simulink model "vd_controller_E9"  (R2017b)
settings: configuration reference "E9_ECU_Configuration" (kept outside this file)
undefined symbols (not defined in the file or in its folder): activate_TC_forMinimal_pTC, ConstantSlipPercent_XCP_pTC, DifferentTorqueFrontAxis_tc, disable_9D_front, disable_9D_rear, disable_slipanglesensor, DiscIntNeverNeededParam, Fz0, lambda_mux_switch_over_XCP_pTC, lambda_mux_XCP_pTC, Lyap_kp_switch_over_XCP_pTC, Lyap_kp_XCP_pTC, Lyap_p, Lyap_TCint, LyapDiscFilter, lyapFilterCoeff_switch_over_XCP_pTC, lyapFilterCoeff_XCP_pTC, mask_SelectInput_pGL, p_Dx1, p_Dx2, Slip_switch_over_XCP_pTC, Sq_PosBadGradient, Sq_PosIsFrozen, Sq_PosOutOfBounds, tire_r_dyn, velLimitInput_switch_over_XCP_pTC, velLimitInput_XCP_pTC, WheelInertia
libraries: SignalProcessingLib x37, simulink x30, hdlsllib x3
(part 1 of 2)
settings Model: DataDictionary=dd_MainControl_E9.sldd  ExplicitPartitioning=on  Creator=chwit  LastModifiedBy=gt-testing
settings Model: ModifiedComment=|
  | schwa -- Fri Mar 02 10:09:33 2018 -- Version 1.53
  | Switched names of ControlAllocation, minimal Version active
settings Model: ModifiedHistory=|
  | schwa -- Fri Mar 02 10:09:33 2018 -- Version 1.53
  | Switched names of ControlAllocation, minimal Version active
  | 
  | schwa -- Fri Mar 02 10:09:33 2018 -- Version 1.53
  | Switched names of ControlAllocation, minimal Version active
  | 
  | schwa -- Fri Mar 02 01:32:20 2018 -- Version 1.52
  | cosmetic changes, adjusted ports
  | 
  | schwa -- Fri Mar 02 01:28:29 2018 -- Version 1.51
  | 
  | schwa -- Fri Mar 02 01:26:02 2018 -- Version 1.50
  | integrated new FF
  | 
  | 
  | chwit -- Fri Feb 23 19:55:57 2018 -- Version 1.49
  | 
  | chwit -- Fri Feb 23 07:06:27 2018 -- Version 1.48
  | Buildable but yet not flashable version of initial version of ControlSystem for E9 after function freeze v1
  | 
  | 
  | 
  | chwit -- Sun Feb 18 18:12:23 2018 -- Version 1.20
  | 
  | chwit -- Sun Feb 18 18:12:23 2018 -- Version 1.20
  | 
  | chwit -- Sun Feb 18 18:02:59 2018 -- Version 1.19
  | 
  | chwit -- Sun Feb 18 17:57:29 2018 -- Version 1.18
  | Saving
  | 
  | 
  | chwit -- Sun Feb 18 17:09:51 2018 -- Version 1.17
  | Saving
  | 
  | chwit -- Sun Feb 18 17:09:04 2018 -- Version 1.16
  | Just for saving purposes
  | 
  | chwit -- Sun Feb 18 14:38:44 2018 -- Version 1.15
  | YawMoment -> YawAcc corrected
  | 
  | 
  | chwit -- Sun Feb 18 12:57:57 2018 -- Version 1.14
  | Function freeze and new structure
  | 
  | 
  | chwit -- Sun Feb 18 12:51:11 2018 -- Version 1.13
  | Changes made due to function freeze and new structure
  | 
  | 
  | chwit -- Sun Feb 18 11:51:16 2018 -- Version 1.11
  | Implemented Manual Mode
  | 
  | chwit -- Sun Feb 18 11:51:16 2018 -- Version 1.11
  | Implemented Manual Mode
  | 
  | Marko -- Sat Feb 17 23:21:38 2018 -- Version 1.10
  | Changed Subsystem ConvertToInverterSingals: Deleted Everything except kt-Kennlinie, added limit on TorqueRequest
  | 
  | added OverUndersteerCorrection between FF and CA, connected CA with temporary (dummy) signals until right signals are provided
  | schwa -- Wed Feb 14 10:07:50 2018 -- Version 1.9
  | 
  | rearranged signals
  | schwa -- Wed Feb 14 09:51:50 2018 -- Version 1.8
  | 
  | chwit -- Sat Jan 20 18:54:27 2018 -- Version 1.7
  | 
  | chwit -- Sat Jan 20 17:46:44 2018 -- Version 1.6
  | 
  | chwit -- Sat Jan 20 17:42:35 2018 -- Version 1.5
  | Initial version
settings ConfigSetRef: DDName=dd_MainControl_E9.sldd

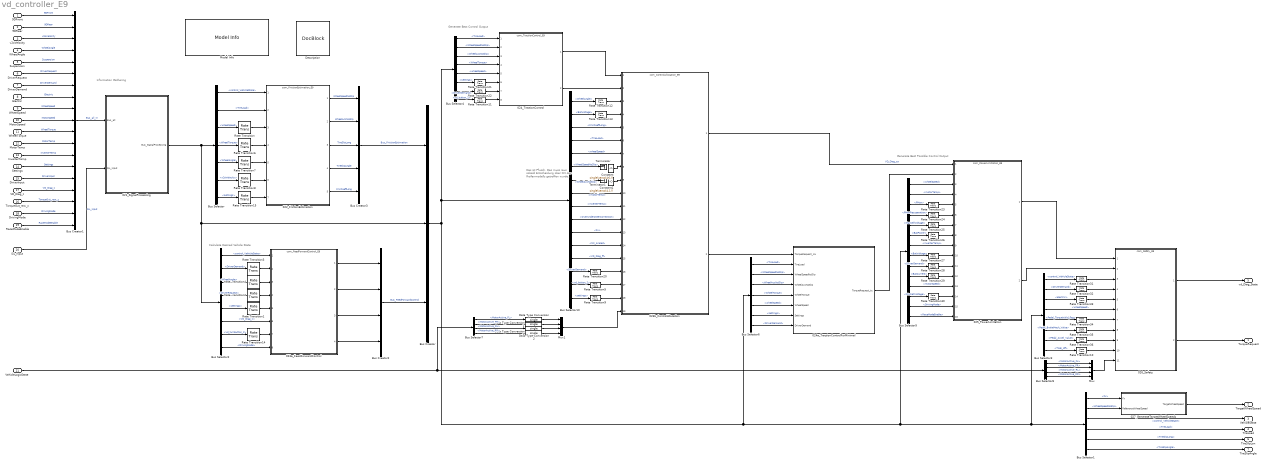
== system vd_controller_E9 ==
  note: Das ist Pfusch.
      | Das muss raus sobald
      | Entscheidung über Ort des
      |  Reifenmodells getroffen wurde.
  note: Information Gathering
  note: Calculate Desired Vehicle State
  note: Generate Best Control Output
  note: Generate Best Possible Control Output
  9DFront : Inport  OutDataTypeStr=Bus: control_9D
  9DRear : Inport  Port=2  OutDataTypeStr=Bus: control_9D
  v2oVelocity : Inport  Port=3  OutDataTypeStr=Bus: control_Velocity  SampleTime=0.004
  WheelAngle : Inport  Port=4  OutDataTypeStr=Bus: control_WheelAngle  SampleTime=0.01
  Suspension : Inport  Port=5  OutDataTypeStr=Bus: control_Suspension  SampleTime=0.01
  DriverRequest : Inport  Port=6  OutDataTypeStr=Bus: control_DriverRequest  SampleTime=0.01
  DriverDemand : Inport  Port=7  OutDataTypeStr=single  PortDimensions=1  SampleTime=0.01
  Electric : Inport  Port=8  OutDataTypeStr=Bus: control_Electric  SampleTime=0.002
  WheelSpeed : Inport  Port=9  OutDataTypeStr=single  PortDimensions=4  SampleTime=0.001
  MotorSpeed : Inport  Port=10  OutDataTypeStr=single  PortDimensions=[4 1]
  WheelTorque : Inport  Port=11  OutDataTypeStr=single  PortDimensions=4  SampleTime=0.001
  MotorTemp : Inport  Port=12  OutDataTypeStr=single  PortDimensions=[4 1]
  InverterTemp : Inport  Port=13  PortDimensions=[4 1]
  Settings : Inport  Port=14  OutDataTypeStr=Bus: control_Settings  SampleTime=0.1
  DriverInput : Inport  Port=15  OutDataTypeStr=Bus: control_DriverInput  SampleTime=0.1
  TorqueOut_raw_z : Inport  Port=16  OutDataTypeStr=single  PortDimensions=4
  VD_Diag_z : Inport  Port=17  OutDataTypeStr=uint16
  DrivingMode : Inport  Port=18  OutDataTypeStr=single  PortDimensions=1
  RaceModeEnable : Inport  Port=19  OutDataTypeStr=boolean
  SiL_Input : Inport  Port=20  OutDataTypeStr=Bus: control_SiL_Input
  VehicleLogicState : Inport  Port=21  OutDataTypeStr=Bus: control_VehicleLogicState
  021_SignalProcessing : Subsystem
  022_FrictionEstimation : ModelReference  ModelNameDialog=com_FrictionEstimation_E9.slx  SimulationMode=Normal  ModelReferenceVersion=1.57
  023a_FeedForwardControl : ModelReference  ModelNameDialog=com_FeedForwardControl_E9.slx  SimulationMode=Normal  ModelReferenceVersion=1.225
  023b_ControlAllocation : ModelReference  ModelNameDialog=com_ControlAllocation_E9.slx  SimulationMode=Normal  ModelReferenceVersion=1.346
  024_TractionControl : ModelReference  ModelNameDialog=com_TractionControl_E9.slx  SimulationMode=Normal  ModelReferenceVersion=1.68
  024a_TractionControlForMinimal : Subsystem
  025_PowerLimitation : ModelReference  ModelNameDialog=com_PowerLimitation_E9.slx  SimulationMode=Normal  ModelReferenceVersion=1.208
  026_Safety : ModelReference  ModelNameDialog=com_Safety_E9.slx  SimulationMode=Normal  ModelReferenceVersion=1.81
  027_GenerateTargetWheelSpeeds : Subsystem
  Bus Creator : BusCreator  Inputs=3
  Bus Creator1 : BusCreator  Inputs=19
  Bus Creator2 : BusCreator  Inputs=4
  Bus Creator3 : BusCreator  Inputs=5
  Bus Selector : BusSelector  OutputSignals=control_VehicleState,TireLoad,wheelSpeed,WheelTorque,WheelAngle,v2oVelocity,settings
  Bus Selector1 : BusSelector  OutputSignals=Bus_FeedForwardControl.Fx,Bus_FrictionEstimation.WheelSpeedNoSlip,Bus_SignalProcessing.control_VehicleState,Bus_SignalProcessing.TireLoad,Bus_FrictionEstimation.TireSlipLong,Bus_FrictionEstimation.TireSlipAngle
  Bus Selector10 : BusSelector  OutputSignals=Bus_SignalProcessing.WheelAngle,Bus_SignalProcessing.electric.BatVoltage,Bus_FrictionEstimation.FricCoeffLong,Bus_SignalProcessing.TireLoad,Bus_SignalProcessing.wheelSpeed,Bus_FrictionEstimation.WheelSpeedNoSlip,Bus_FrictionEstimation.WheelAccNoSlip,Bus_SignalProcessing.motorTemp,Bus_SignalProcessing.inverterTemp,Bus_FeedForwardControl.OverUndersteerCorrection,Bus_FeedForwardControl.Fx,Bus_FeedForwardControl.Mz_scaled,Bus_FeedForwardControl.VD_Diag_ff,Bus_SignalProcessing.DriverDemand,Bus_SignalProcessing.HMI_DriverNotice.vd_button_2,Bus_SignalProcessing.settings
  Bus Selector2 : BusSelector  OutputSignals=control_VehicleState,DriverDemand,WheelAngle,DriverRequest,settings,VD_Diag_z,HMI_DriverNotice.vd_turnbutton_2,HMI_DriverNotice.DrivingMode
  Bus Selector3 : BusSelector  OutputSignals=Bus_SignalProcessing.control_VehicleState,Bus_SignalProcessing.DriverDemand,Bus_SignalProcessing.electric,Bus_SignalProcessing.wheelSpeed,Bus_SignalProcessing.DriverRequest.Pedal_TorqueValid_flag,Bus_SignalProcessing.DriverRequest.Pedal_BrakeMech_Value,Bus_SignalProcessing.DriverRequest.Pedal_Accel_Value,Bus_SignalProcessing.settings.TWB_off
  Bus Selector4 : BusSelector  OutputSignals=Bus_SignalProcessing.TireLoad,Bus_FrictionEstimation.WheelSpeedNoSlip,Bus_FrictionEstimation.WheelAccNoSlip,Bus_SignalProcessing.WheelTorque,Bus_SignalProcessing.wheelSpeed,Bus_SignalProcessing.settings,Bus_SignalProcessing.DriverDemand,Bus_SignalProcessing.HMI_DriverNotice.vd_button_2
  Bus Selector5 : BusSelector  OutputSignals=Bus_SignalProcessing.wheelSpeed,Bus_SignalProcessing.motorTemp,Bus_SignalProcessing.settings.PMax,Bus_SignalProcessing.settings.PMaxRecuperation,Bus_SignalProcessing.electric.MaxCellVoltage,Bus_SignalProcessing.electric.BatPower,Bus_SignalProcessing.inverterTemp,Bus_SignalProcessing.electric.BatVoltage,Bus_SignalProcessing.DriverDemand,Bus_SignalProcessing.electric.BatCurrent,Bus_SignalProcessing.motorSpeed,Bus_SignalProcessing.electric.MinCellVoltage,Bus_SignalProcessing.HMI_DriverNotice.DrivingMode,Bus_SignalProcessing.RaceModeEnable
  Bus Selector6 : BusSelector  OutputSignals=Bus_SignalProcessing.TireLoad,Bus_FrictionEstimation.WheelSpeedNoSlip,Bus_FrictionEstimation.WheelAccNoSlip,Bus_SignalProcessing.WheelTorque,Bus_SignalProcessing.wheelSpeed,Bus_SignalProcessing.settings,Bus_SignalProcessing.DriverDemand
  Bus Selector7 : BusSelector  OutputSignals=MotorActive_FL,MotorActive_FR,MotorActive_RL,MotorActive_RR
  Bus Selector8 : BusSelector  OutputSignals=MotorActive_FL,MotorActive_FR,MotorActive_RL,MotorActive_RR
  Constant : Constant  Value=single(zeros(4,1))
  Constant1 : Constant  Value=single(zeros(4,1))
  Data Type Conversion{,1..3} (4 alike) : DataTypeConversion  OutDataTypeStr=single
  Description : simulink/Model-Wide Utilities/DocBlock  DocumentType=Text
      content=|
      | Beschreibung:
      |
      | Schlupfsollwert wird über Settings-Protokoll vorgegeben. Wird entsprechend mit Vorzeichen Torque-Request verrechnet.
      | Desgin-Parameter sind Lyap_kp (nützlich, linearer Faktor) und Lyap_p (nicht so nützlich, Potenz -> sollte ungerade sein (nicht ganz sicher)).
      |
      | I-Anteil mit Anti-WindUp zur Verbesserung Regler und Stellgrößenbeschränkung vorzubeugen.
      |
      | Tiefpassfilter (PT1) zur Verminderung von Schwingungen.
      |
      | Lambda_mux ist der Einstellparameter für den Reibwert, mit dem das SetUp stark verändert werden kann.
      |
      | Multiport-Switches zur Auswahl diverser Ansätze für die Traktionskontrolle bzw. zur Abschaltung.
      |
      | Adaptive_RG Schlupfgeschw.: adaptiver Regler mit Reibwerschätzer, schätzt Reibwert und regelt entsprechend Schlupf
      |     -> hat nicht wirklich funktioniert, Schätzen war wohl schon scheiße, Konzept fragwürdig
      |
      | LQRI: Linearisierter Lyap. Regler mit diversen Betriebspunkten (Gain-Scheduling), ähnliche Gleichungen wie Lyap
      |     -> durch Linearisierung etwas schlechter als Lyap
  Model Info : simulink/Model-Wide Utilities/Model Info  Frame=on  DisplayStringWithTags=|  HorizontalTextAlignment=Center  LeftAlignmentValue=0.5
      | Model Name: %<ModelName>
      | Responsible: Christian Witte
      | 
      | Last modified by: %<LastModifiedBy>
      | Last modified: %<LastModificationDate>
      | Current Version: %<ModelVersion>
  Mux : Mux
  Mux1 : Mux
  Rate Transition{,1..4,6..8,14..15} (10 alike) : RateTransition  Deterministic=off  OutPortSampleTime=0.002
  Rate Transition{5,9..13,20..36} (23 alike) : RateTransition  Deterministic=off  OutPortSampleTime=0.001
  Terminator : Terminator
  Terminator1 : Terminator
  TorqueRequest : Outport  OutDataTypeStr=single  PortDimensions=4
  TargetWheelSpeed : Outport  Port=2  OutDataTypeStr=single  PortDimensions=4
  VehicleState : Outport  Port=3  OutDataTypeStr=Bus: control_VehicleState
  TireLoad : Outport  Port=4  SignalName=TireLoad  OutDataTypeStr=single  PortDimensions=4
  vd_Diag_State : Outport  Port=5  OutDataTypeStr=uint16
  TireSlipLon : Outport  Port=6  OutDataTypeStr=single  PortDimensions=4
  TireSlipAngle : Outport  Port=7  OutDataTypeStr=single  PortDimensions=4
  wires:
  022_FrictionEstimation/3 -> Bus Creator3/3  "TireSlipLong"
  Bus Selector/2 -> 022_FrictionEstimation/2  "<TireLoad>"
  022_FrictionEstimation/2 -> Bus Creator3/2  "WheelAccNoSlip"
  Bus Selector/3 -> Rate Transition/1  "<wheelSpeed>"
  Bus Selector/1 -> 022_FrictionEstimation/1  "<control_VehicleState>"
  022_FrictionEstimation/1 -> Bus Creator3/1  "WheelSpeedNoSlip"
  Bus Creator3/1 -> Bus Creator/1  "Bus_FrictionEstimation"
  022_FrictionEstimation/4 -> Bus Creator3/4  "TireSlipAngle"
  025_PowerLimitation/1 -> 026_Safety/1
  023a_FeedForwardControl/4 -> Bus Creator2/4
  023b_ControlAllocation/1 -> 025_PowerLimitation/1  "VD_Diag_ca"
  Bus Creator1/1 -> 021_SignalProcessing/1(Bus_all)  "Bus_all_in"
  Bus Creator2/1 -> Bus Creator/3  "Bus_FeedForwardControl"
  021_SignalProcessing/1(Bus_SignalProcessing) -> Bus Selector/1, Bus Creator/2, Bus Selector2/1
  023a_FeedForwardControl/1 -> Bus Creator2/1
  023a_FeedForwardControl/3 -> Bus Creator2/3
  022_FrictionEstimation/5 -> Bus Creator3/5  "FricCoeffLong"
  Bus Creator/1 -> Bus Selector10/1, Bus Selector4/1, Bus Selector6/1, Bus Selector5/1, Bus Selector3/1, Bus Selector1/1
  Bus Selector1/3 -> VehicleState/1  "<control_VehicleState>"
  Bus Selector1/4 -> TireLoad/1  "<TireLoad>"
  023a_FeedForwardControl/2 -> Bus Creator2/2
  023b_ControlAllocation/2 -> 024a_TractionControlForMinimal/1(TorqueRequest_ca)
  Bus Selector5/1 -> 025_PowerLimitation/3  "<wheelSpeed>"
  Bus Selector5/2 -> 025_PowerLimitation/4  "<motorTemp>"
  Bus Selector5/3 -> Rate Transition23/1  "<PMax>"
  Bus Selector5/4 -> Rate Transition24/1  "<PMaxRecuperation>"
  Bus Selector5/5 -> Rate Transition25/1  "<MaxCellVoltage>"
  Bus Selector5/6 -> Rate Transition26/1  "<BatPower>"
  Bus Selector5/7 -> 025_PowerLimitation/9  "<inverterTemp>"
  Bus Selector5/8 -> Rate Transition27/1  "<BatVoltage>"
  Bus Selector5/9 -> Rate Transition28/1  "<DriverDemand>"
  Bus Selector3/1 -> Rate Transition31/1  "<control_VehicleState>"
  Bus Selector3/2 -> Rate Transition32/1  "<DriverDemand>"
  Bus Selector3/3 -> Rate Transition33/1  "<electric>"
  Bus Selector3/4 -> 026_Safety/6  "<wheelSpeed>"
  Bus Selector3/5 -> Rate Transition34/1  "<Pedal_TorqueValid_flag>"
  025_PowerLimitation/2 -> 026_Safety/2
  Bus Selector10/1 -> Rate Transition12/1  "<WheelAngle>"
  Bus Selector10/2 -> Rate Transition13/1  "<BatVoltage>"
  Bus Selector10/3 -> 023b_ControlAllocation/5  "<FricCoeffLong>"
  Bus Selector10/4 -> 023b_ControlAllocation/6  "<TireLoad>"
  Bus Selector10/5 -> 023b_ControlAllocation/7  "<wheelSpeed>"
  Bus Selector10/8 -> 023b_ControlAllocation/10  "<motorTemp>"
  Bus Selector10/9 -> 023b_ControlAllocation/11  "<inverterTemp>"
  Bus Selector10/10 -> 023b_ControlAllocation/12  "<OverUndersteerCorrection>"
  Bus Selector10/11 -> 023b_ControlAllocation/13  "<Fx>"
  026_Safety/2 -> TorqueRequest/1
  026_Safety/1 -> vd_Diag_State/1
  Bus Selector4/7 -> Rate Transition22/1  "<DriverDemand>"
  Bus Selector4/6 -> Rate Transition21/1  "<settings>"
  Bus Selector4/5 -> 024_TractionControl/5  "<wheelSpeed>"
  Bus Selector4/4 -> 024_TractionControl/4  "<WheelTorque>"
  Bus Selector4/3 -> 024_TractionControl/3  "<WheelAccNoSlip>"
  Bus Selector4/2 -> 024_TractionControl/2  "<WheelSpeedNoSlip>"
  Bus Selector4/1 -> 024_TractionControl/1  "<TireLoad>"
  Bus Selector10/13 -> 023b_ControlAllocation/15  "<VD_Diag_ff>"
  024_TractionControl/2 -> 023b_ControlAllocation/2
  024_TractionControl/1 -> 023b_ControlAllocation/1
  Constant/1 -> 023b_ControlAllocation/8
  Constant1/1 -> 023b_ControlAllocation/9
  Bus Selector10/6 -> Terminator/1  "<WheelSpeedNoSlip>"
  Bus Selector10/7 -> Terminator1/1  "<WheelAccNoSlip>"
  Bus Selector/4 -> Rate Transition6/1  "<WheelTorque>"
  Bus Selector/5 -> Rate Transition7/1  "<WheelAngle>"
  Bus Selector/6 -> Rate Transition8/1  "<v2oVelocity>"
  9DFront/1 -> Bus Creator1/1  "9DFront"
  9DRear/1 -> Bus Creator1/2  "9DRear"
  v2oVelocity/1 -> Bus Creator1/3  "v2oVelocity"
  WheelAngle/1 -> Bus Creator1/4  "WheelAngle"
  Suspension/1 -> Bus Creator1/5  "Suspension"
  DriverRequest/1 -> Bus Creator1/6  "DriverRequest"
  DriverDemand/1 -> Bus Creator1/7  "DriverDemand"
  TorqueOut_raw_z/1 -> Bus Creator1/17  "TorqueOut_raw_z"
  Electric/1 -> Bus Creator1/8  "Electric"
  VD_Diag_z/1 -> Bus Creator1/16  "VD_Diag_z"
  WheelSpeed/1 -> Bus Creator1/9  "WheelSpeed"
  MotorSpeed/1 -> Bus Creator1/10  "MotorSpeed"
  WheelTorque/1 -> Bus Creator1/11  "WheelTorque"
  MotorTemp/1 -> Bus Creator1/12  "MotorTemp"
  InverterTemp/1 -> Bus Creator1/13  "InverterTemp"
  Settings/1 -> Bus Creator1/14  "Settings"
  DriverInput/1 -> Bus Creator1/15  "DriverInput"
  Bus Selector2/1 -> 023a_FeedForwardControl/1  "<control_VehicleState>"
  Bus Selector2/2 -> Rate Transition3/1  "<DriverDemand>"
  Bus Selector2/3 -> Rate Transition4/1  "<WheelAngle>"
  Bus Selector2/4 -> Rate Transition2/1  "<DriverRequest>"
  Bus Selector2/5 -> Rate Transition1/1  "<settings>"
  Bus Selector2/6 -> 023a_FeedForwardControl/6  "<VD_Diag_z>"
  Bus Selector5/10 -> Rate Transition29/1  "<BatCurrent>"
  Bus Selector3/6 -> Rate Transition35/1  "<Pedal_BrakeMech_Value>"
  Bus Selector3/7 -> Rate Transition36/1  "<Pedal_Accel_Value>"
  SiL_Input/1 -> 021_SignalProcessing/2(SiL_Input)  "SiL_Input"
  Bus Selector10/14 -> Rate Transition20/1  "<DriverDemand>"
  Bus Selector1/2 -> 027_GenerateTargetWheelSpeeds/2(ReferenceWheelSpeed)  "<WheelSpeedNoSlip>"
  027_GenerateTargetWheelSpeeds/1(TargetWheelSpeed) -> TargetWheelSpeed/1
  Bus Selector1/1 -> 027_GenerateTargetWheelSpeeds/1(Fx)  "<Fx>"
  024a_TractionControlForMinimal/1(TorqueRequest_tc) -> 025_PowerLimitation/2
  Bus Selector6/1 -> 024a_TractionControlForMinimal/2(TireLoad)  "<TireLoad>"
  Bus Selector6/2 -> 024a_TractionControlForMinimal/3(WheelSpeedNoSlip)  "<WheelSpeedNoSlip>"
  Bus Selector6/3 -> 024a_TractionControlForMinimal/4(WheelAccNoSlip)  "<WheelAccNoSlip>"
  Bus Selector6/4 -> 024a_TractionControlForMinimal/5(WheelTorque)  "<WheelTorque>"
  Bus Selector6/5 -> 024a_TractionControlForMinimal/6(WheelSpeed)  "<wheelSpeed>"
  Bus Selector6/6 -> 024a_TractionControlForMinimal/7(Settings)  "<settings>"
  Bus Selector6/7 -> 024a_TractionControlForMinimal/8(DriverDemand)  "<DriverDemand>"
  Bus Selector5/11 -> 025_PowerLimitation/13  "<motorSpeed>"
  VehicleLogicState/1 -> Bus Selector7/1, Bus Selector8/1
  Rate Transition4/1 -> 023a_FeedForwardControl/3
  Rate Transition1/1 -> 023a_FeedForwardControl/5
  Rate Transition2/1 -> 023a_FeedForwardControl/4
  Rate Transition3/1 -> 023a_FeedForwardControl/2
  Rate Transition/1 -> 022_FrictionEstimation/3
  Rate Transition6/1 -> 022_FrictionEstimation/4
  Rate Transition7/1 -> 022_FrictionEstimation/5
  Rate Transition8/1 -> 022_FrictionEstimation/6
  Rate Transition12/1 -> 023b_ControlAllocation/3
  Rate Transition13/1 -> 023b_ControlAllocation/4
  Rate Transition20/1 -> 023b_ControlAllocation/16
  Rate Transition21/1 -> 024_TractionControl/6
  Rate Transition22/1 -> 024_TractionControl/7
  Rate Transition23/1 -> 025_PowerLimitation/5
  Rate Transition24/1 -> 025_PowerLimitation/6
  Rate Transition26/1 -> 025_PowerLimitation/8
  Rate Transition25/1 -> 025_PowerLimitation/7
  Rate Transition27/1 -> 025_PowerLimitation/10
  Rate Transition28/1 -> 025_PowerLimitation/11
  Rate Transition29/1 -> 025_PowerLimitation/12
  Rate Transition30/1 -> 025_PowerLimitation/14
  Rate Transition31/1 -> 026_Safety/3
  Rate Transition32/1 -> 026_Safety/4
  Rate Transition33/1 -> 026_Safety/5
  Rate Transition34/1 -> 026_Safety/7
  Rate Transition35/1 -> 026_Safety/8
  Rate Transition36/1 -> 026_Safety/9
  Bus Selector8/1 -> Mux/1  "<MotorActive_FL>"
  Bus Selector8/2 -> Mux/2  "<MotorActive_FR>"
  Bus Selector8/3 -> Mux/3  "<MotorActive_RL>"
  Bus Selector8/4 -> Mux/4  "<MotorActive_RR>"
  Mux/1 -> 026_Safety/11
  DrivingMode/1 -> Bus Creator1/18  "DrivingMode"
  Bus Selector5/13 -> 025_PowerLimitation/15  "<DrivingMode>"
  Bus Selector5/12 -> Rate Transition30/1  "<MinCellVoltage>"
  Bus Selector4/8 -> Rate Transition11/1  "<vd_button_2>"
  Rate Transition11/1 -> 024_TractionControl/8
  Bus Selector7/4 -> Data Type Conversion3/1  "<MotorActive_RR>"
  Mux1/1 -> 023b_ControlAllocation/19
  Bus Selector7/1 -> Data Type Conversion/1  "<MotorActive_FL>"
  Bus Selector7/2 -> Data Type Conversion1/1  "<MotorActive_FR>"
  Bus Selector7/3 -> Data Type Conversion2/1  "<MotorActive_RL>"
  Data Type Conversion/1 -> Mux1/1
  Data Type Conversion1/1 -> Mux1/2
  Data Type Conversion2/1 -> Mux1/3
  Data Type Conversion3/1 -> Mux1/4
  Bus Selector1/5 -> TireSlipLon/1  "<TireSlipLong>"
  Bus Selector1/6 -> TireSlipAngle/1  "<TireSlipAngle>"
  Bus Selector2/7 -> Rate Transition14/1  "<vd_turnbutton_2>"
  Rate Transition14/1 -> 023a_FeedForwardControl/7
  Bus Selector/7 -> Rate Transition15/1  "<settings>"
  Rate Transition15/1 -> 022_FrictionEstimation/7
  Bus Selector10/15 -> Rate Transition5/1  "<vd_button_2>"
  Rate Transition5/1 -> 023b_ControlAllocation/17
  Bus Selector10/16 -> Rate Transition9/1  "<settings>"
  Rate Transition9/1 -> 023b_ControlAllocation/18
  Bus Selector2/8 -> 023a_FeedForwardControl/8  "<DrivingMode>"
  RaceModeEnable/1 -> Bus Creator1/19  "RaceModeEnable"
  Bus Selector5/14 -> 025_PowerLimitation/16  "<RaceModeEnable>"
  Bus Selector3/8 -> Rate Transition10/1  "<TWB_off>"
  Rate Transition10/1 -> 026_Safety/10
  Bus Selector10/12 -> 023b_ControlAllocation/14  "<Mz_scaled>"

== system vd_controller_E9/021_SignalProcessing ==
  Bus_all : Inport
  SiL_Input : Inport  Port=2
  211_SensorFusion : ModelReference  ModelNameDialog=com_SensorFusion.slx  SimulationMode=Normal  ModelReferenceVersion=1.119
  212_ManualMode : Subsystem
  213_PlausibiltyCheckandSignalMatching : Subsystem
  Bus Creator : BusCreator  Inputs=2
  Bus Selector : BusSelector  OutputSignals=9DFront,9DRear,v2oVelocity,WheelSpeed,Suspension,WheelTorque,WheelAngle
  Rate Transition{,1..4} (5 alike) : RateTransition
  Bus_SignalProcessing : Outport
  wires:
  211_SensorFusion/2 -> Bus Creator/2  "TireLoad"
  211_SensorFusion/1 -> Bus Creator/1
  212_ManualMode/1(Bus_SignalProcessing) -> Bus_SignalProcessing/1  "Bus_SignalProcessing"
  Bus Creator/1 -> 212_ManualMode/1(Bus_SensorFusion)  "Bus_Sensorfusion"
  Bus_all/1 -> 213_PlausibiltyCheckandSignalMatching/1(Bus_all)
  Bus Selector/5 -> Rate Transition2/1  "<Suspension>"
  Bus Selector/2 -> 211_SensorFusion/2  "<9DRear>"
  Bus Selector/3 -> Rate Transition4/1  "<v2oVelocity>"
  Bus Selector/1 -> 211_SensorFusion/1  "<9DFront>"
  Bus Selector/4 -> Rate Transition3/1  "<WheelSpeed>"
  Bus Selector/6 -> Rate Transition1/1  "<WheelTorque>"
  Bus Selector/7 -> Rate Transition/1  "<WheelAngle>"
  213_PlausibiltyCheckandSignalMatching/1(Bus_SignalProcessing) -> 212_ManualMode/2(Bus_all), Bus Selector/1
  SiL_Input/1 -> 212_ManualMode/3(SiL_Input)
  Rate Transition/1 -> 211_SensorFusion/7
  Rate Transition1/1 -> 211_SensorFusion/6
  Rate Transition2/1 -> 211_SensorFusion/5
  Rate Transition3/1 -> 211_SensorFusion/4
  Rate Transition4/1 -> 211_SensorFusion/3

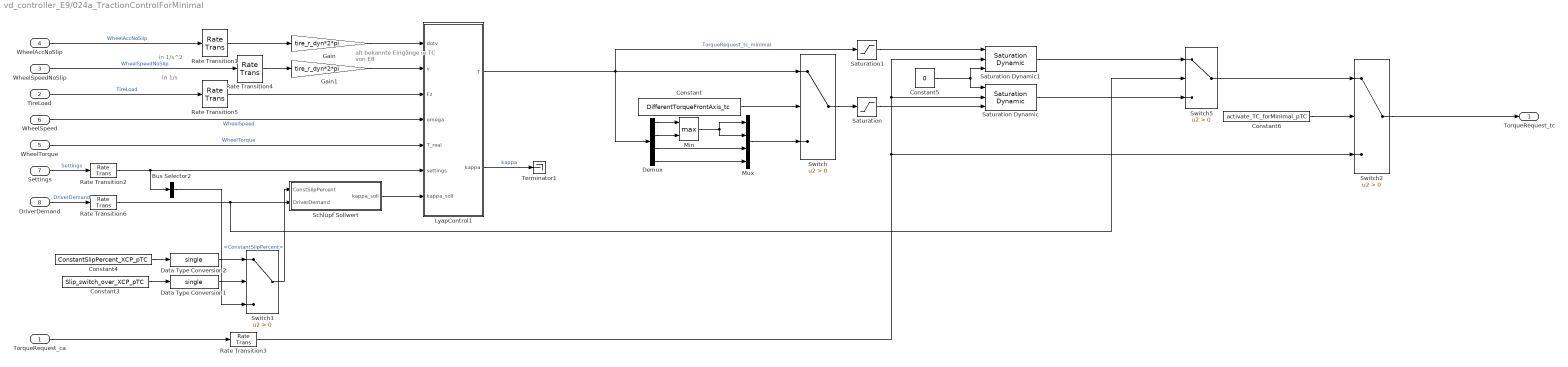
== system vd_controller_E9/024a_TractionControlForMinimal ==
  note: in 1/s
  note: alt bekannte Eingänge
      | in TC von E8
  note: in 1/s^2
  TorqueRequest_ca : Inport  OutDataTypeStr=single  PortDimensions=4
  TireLoad : Inport  Port=2  OutDataTypeStr=single  PortDimensions=4
  WheelSpeedNoSlip : Inport  Port=3  OutDataTypeStr=single  PortDimensions=4
  WheelAccNoSlip : Inport  Port=4  OutDataTypeStr=single  PortDimensions=4
  WheelTorque : Inport  Port=5  OutDataTypeStr=single  PortDimensions=4
  WheelSpeed : Inport  Port=6  OutDataTypeStr=single  PortDimensions=4
  Settings : Inport  Port=7
  DriverDemand : Inport  Port=8  OutDataTypeStr=single
  Bus Selector2 : BusSelector  OutputSignals=ConstantSlipPercent
  Constant : Constant  Value=DifferentTorqueFrontAxis_tc  OutDataTypeStr=boolean
  Constant3 : Constant  Value=Slip_switch_over_XCP_pTC
  Constant4 : Constant  Value=ConstantSlipPercent_XCP_pTC
  Constant5 : Constant  Value=0  OutDataTypeStr=single
  Constant6 : Constant  Value=activate_TC_forMinimal_pTC
  Data Type Conversion1 : DataTypeConversion  OutDataTypeStr=single
  Data Type Conversion2 : DataTypeConversion  OutDataTypeStr=single
  Demux : Demux
  Gain : Gain  Gain=tire_r_dyn*2*pi
  Gain1 : Gain  Gain=tire_r_dyn*2*pi
  LyapControl1 : Subsystem
  Min : MinMax  Function=max  Inputs=2
  Mux : Mux
  Rate Transition{1..2,4..6} (5 alike) : RateTransition  Deterministic=off  OutPortSampleTime=0.001
  Rate Transition3 : RateTransition  OutPortSampleTime=0.001
  Saturation : Saturate  UpperLimit=0  LowerLimit=-inf
  Saturation Dynamic : simulink/Discontinuities/Saturation Dynamic  OutMin=[]  OutMax=[]  OutDataTypeStr=Inherit: Same as second input  OutDataType=fixdt(1, 16)  OutScaling=2^-10  DoSatur=off
  Saturation Dynamic1 : simulink/Discontinuities/Saturation Dynamic  OutMin=[]  OutMax=[]  OutDataTypeStr=Inherit: Same as second input  OutDataType=fixdt(1, 16)  OutScaling=2^-10  DoSatur=off
  Saturation1 : Saturate  UpperLimit=inf  LowerLimit=0
  Schlupf Sollwert : Subsystem
  Switch : Switch  Criteria=u2 > Threshold
  Switch1 : Switch  Criteria=u2 > Threshold
  Switch2 : Switch  Criteria=u2 > Threshold
  Switch5 : Switch  Criteria=u2 > Threshold  OutDataTypeStr=single
  Terminator1 : Terminator
  TorqueRequest_tc : Outport
  wires:
  Bus Selector2/1 -> Switch1/3  "<ConstantSlipPercent>"
  Switch1/1 -> Schlupf Sollwert/1(ConstSlipPercent)
  Data Type Conversion2/1 -> Switch1/1
  Constant3/1 -> Data Type Conversion1/1
  Rate Transition4/1 -> Gain1/1
  Data Type Conversion1/1 -> Switch1/2
  Rate Transition1/1 -> Gain/1
  Schlupf Sollwert/1(kappa_soll) -> LyapControl1/7(kappa_soll)
  Constant4/1 -> Data Type Conversion2/1
  WheelTorque/1 -> LyapControl1/5(T_real)  "WheelTorque"
  LyapControl1/1(T) -> Saturation1/1, Switch/1, Demux/1  "TorqueRequest_tc_minimal"
  WheelSpeed/1 -> LyapControl1/4(omega)  "WheelSpeed"
  TireLoad/1 -> Rate Transition5/1  "TireLoad"
  WheelSpeedNoSlip/1 -> Rate Transition4/1  "WheelSpeedNoSlip"
  Gain1/1 -> LyapControl1/2(v)
  Settings/1 -> Rate Transition2/1  "Settings"
  DriverDemand/1 -> Rate Transition6/1  "DriverDemand"
  Gain/1 -> LyapControl1/1(dotv)
  WheelAccNoSlip/1 -> Rate Transition1/1  "WheelAccNoSlip"
  Constant5/1 -> Saturation Dynamic1/3, Saturation Dynamic/1
  TorqueRequest_ca/1 -> Rate Transition3/1
  Saturation Dynamic1/1 -> Switch5/1
  Saturation Dynamic/1 -> Switch5/3
  Switch5/1 -> Switch2/1
  Switch2/1 -> TorqueRequest_tc/1
  LyapControl1/2(kappa) -> Terminator1/1  "kappa"
  Demux/3 -> Mux/3
  Demux/4 -> Mux/4
  Demux/2 -> Min/2
  Min/1 -> Mux/2, Mux/1
  Demux/1 -> Min/1
  Switch/1 -> Saturation/1
  Mux/1 -> Switch/3
  Constant/1 -> Switch/2
  Saturation/1 -> Saturation Dynamic/3
  Saturation1/1 -> Saturation Dynamic1/1
  Rate Transition2/1 -> LyapControl1/6(settings), Bus Selector2/1
  Rate Transition3/1 -> Saturation Dynamic/2, Saturation Dynamic1/2, Switch2/3
  Rate Transition5/1 -> LyapControl1/3(Fz)
  Rate Transition6/1 -> Switch5/2, Schlupf Sollwert/2("DriverDemand ")
  Constant6/1 -> Switch2/2

== system vd_controller_E9/027_GenerateTargetWheelSpeeds ==
  Fx : Inport
  ReferenceWheelSpeed : Inport  Port=2
  Gain : Gain  Gain=0.9
  Gain1 : Gain  Gain=1.1
  Rate Transition2 : RateTransition  Deterministic=off
  Switch : Switch  Criteria=u2 > Threshold
  TargetWheelSpeed : Outport  PortDimensions=4
  wires:
  ReferenceWheelSpeed/1 -> Gain1/1, Gain/1
  Fx/1 -> Rate Transition2/1
  Gain/1 -> Switch/3
  Gain1/1 -> Switch/1
  Switch/1 -> TargetWheelSpeed/1  "TargetWheelSpeed"
  Rate Transition2/1 -> Switch/2

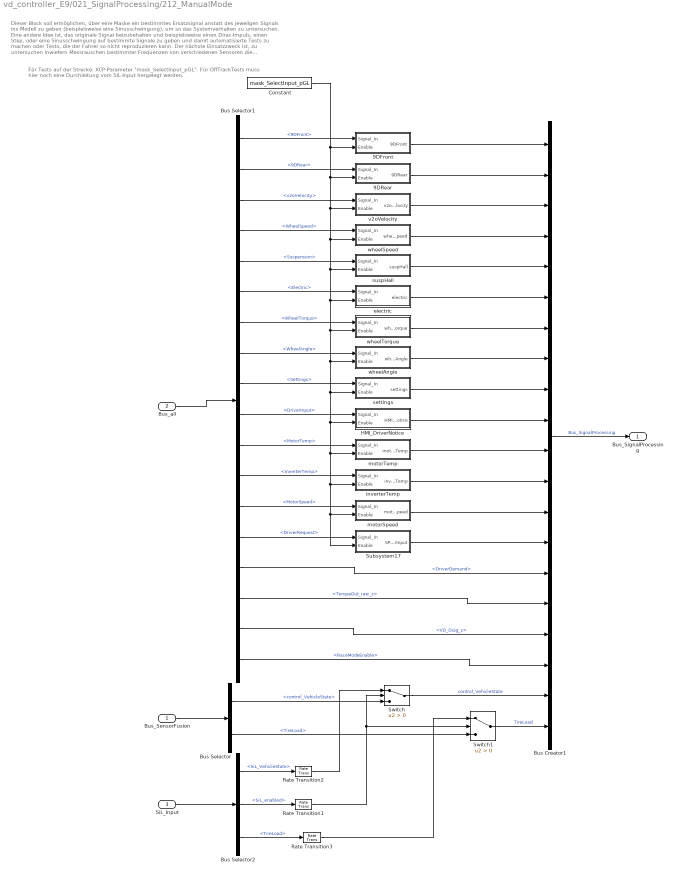
== system vd_controller_E9/021_SignalProcessing/212_ManualMode ==
  note: Für Tests auf der Strecke: XCP-Parameter "mask_SelectInput_pGL".
      | Für OffTrackTests muss hier noch eine Durchleitung vom SiL-Input hergelegt werden.
  note: Dieser Block soll ermöglichen, über eine Maske ein bestimmtes Ersatzsignal anstatt des jeweilgen Signals ins Modell zu geben (beispielsweise eine Sinusschwingung), um so das Systemverhalten zu untersuchen.
      | Eine andere Idee ist, das originale Signal beizubehalten und beispielsweise einen Dirac-Impuls, einen Step, oder eine Sinusschwingung auf bestimmte Signale zu geben und damit automatisierte Tests zu machen oder Tests, die der Fahrer so nicht reproduzieren kann.
      | Der nächste Einsatzzweck ist, zu untersuchen inwiefern Messrauschen bestimmter Frequenzen von verschiedenen Sensoren die Momentenverteilung und den Momentenverlauf beeinflussen.
      | Hier können auch SiSO-Übertragungsfunktionen von den ausgewählten Sensoriksignalen auf die einzelnen Raddrehmomente gebildet werden. Idealerweise fallen diese dann zu hohen Frequenzen hin schnell ab, um keine Fahrzeugschwingungen zu induzieren.
  Bus_SensorFusion : Inport
  Bus_all : Inport  Port=2
  SiL_Input : Inport  Port=3
  9DFront : Subsystem
  9DRear : Subsystem
  Bus Creator1 : BusCreator  Inputs=20
  Bus Selector : BusSelector  OutputSignals=control_VehicleState,TireLoad
  Bus Selector1 : BusSelector  OutputSignals=9DFront,9DRear,v2oVelocity,WheelSpeed,Suspension,Electric,WheelTorque,WheelAngle,Settings,DriverInput,MotorTemp,InverterTemp,MotorSpeed,DriverRequest,DriverDemand,TorqueOut_raw_z,VD_Diag_z,RaceModeEnable
  Bus Selector2 : BusSelector  OutputSignals=SiL_VehicleState,SiL_enabled,TireLoad
  Constant : Constant  Value=mask_SelectInput_pGL
  HMI_DriverNotice : Subsystem
  Rate Transition1 : RateTransition  Deterministic=off  OutPortSampleTime=0.002
  Rate Transition2 : RateTransition  Deterministic=off  OutPortSampleTime=0.002
  Rate Transition3 : RateTransition  Deterministic=off  OutPortSampleTime=0.002
  Subsystem17 : Subsystem
  Switch : Switch  Criteria=u2 > Threshold
  Switch1 : Switch  Criteria=u2 > Threshold
  electric : Subsystem
  inverterTemp : Subsystem
  motorSpeed : Subsystem
  motorTemp : Subsystem
  settings : Subsystem
  suspHall : Subsystem
  v2oVelocity : Subsystem
  wheelAngle : Subsystem
  wheelSpeed : Subsystem
  wheelTorque : Subsystem
  Bus_SignalProcessing : Outport
  wires:
  Bus_SensorFusion/1 -> Bus Selector/1
  settings/1(settings) -> Bus Creator1/9
  wheelAngle/1(wheelAngle) -> Bus Creator1/8
  wheelTorque/1(wheelTorque) -> Bus Creator1/7
  electric/1(electric) -> Bus Creator1/6
  suspHall/1(suspHall) -> Bus Creator1/5
  wheelSpeed/1(wheelSpeed) -> Bus Creator1/4
  v2oVelocity/1(v2oVelocity) -> Bus Creator1/3
  9DRear/1(9DRear) -> Bus Creator1/2
  9DFront/1(9DFront) -> Bus Creator1/1
  Constant/1 -> v2oVelocity/2(Enable), suspHall/2(Enable), Subsystem17/2(Enable), motorSpeed/2(Enable), inverterTemp/2(Enable), motorTemp/2(Enable), HMI_DriverNotice/2(Enable), settings/2(Enable), wheelAngle/2(Enable), wheelTorque/2(Enable), electric/2(Enable), wheelSpeed/2(Enable), 9DRear/2(Enable), 9DFront/2(Enable)
  Bus Selector1/14 -> Subsystem17/1(Signal_In)  "<DriverRequest>"
  Bus Selector1/11 -> motorTemp/1(Signal_In)  "<MotorTemp>"
  Bus Selector1/12 -> inverterTemp/1(Signal_In)  "<InverterTemp>"
  Bus Selector1/13 -> motorSpeed/1(Signal_In)  "<MotorSpeed>"
  Bus Selector1/4 -> wheelSpeed/1(Signal_In)  "<WheelSpeed>"
  Bus Selector1/3 -> v2oVelocity/1(Signal_In)  "<v2oVelocity>"
  Bus_all/1 -> Bus Selector1/1
  Bus Selector1/7 -> wheelTorque/1(Signal_In)  "<WheelTorque>"
  Bus Selector1/10 -> HMI_DriverNotice/1(Signal_In)  "<DriverInput>"
  Bus Selector1/1 -> 9DFront/1(Signal_In)  "<9DFront>"
  Bus Creator1/1 -> Bus_SignalProcessing/1  "Bus_SignalProcessing"
  Bus Selector1/9 -> settings/1(Signal_In)  "<Settings>"
  Bus Selector1/2 -> 9DRear/1(Signal_In)  "<9DRear>"
  Bus Selector1/8 -> wheelAngle/1(Signal_In)  "<WheelAngle>"
  Bus Selector1/5 -> suspHall/1(Signal_In)  "<Suspension>"
  Bus Selector1/6 -> electric/1(Signal_In)  "<Electric>"
  HMI_DriverNotice/1(HMI_DriverNotice) -> Bus Creator1/10
  motorTemp/1(motorTemp) -> Bus Creator1/11
  inverterTemp/1(inverterTemp) -> Bus Creator1/12
  motorSpeed/1(motorSpeed) -> Bus Creator1/13
  Subsystem17/1(SP_DriverInput) -> Bus Creator1/14
  Bus Selector1/15 -> Bus Creator1/15  "<DriverDemand>"
  Bus Selector1/16 -> Bus Creator1/16  "<TorqueOut_raw_z>"
  Bus Selector1/17 -> Bus Creator1/17  "<VD_Diag_z>"
  Bus Selector/1 -> Switch/3  "<control_VehicleState>"
  Bus Selector/2 -> Switch1/3  "<TireLoad>"
  SiL_Input/1 -> Bus Selector2/1
  Bus Selector2/2 -> Rate Transition1/1  "<SiL_enabled>"
  Bus Selector2/1 -> Rate Transition2/1  "<SiL_VehicleState>"
  Bus Selector2/3 -> Rate Transition3/1  "<TireLoad>"
  Switch/1 -> Bus Creator1/19  "control_VehicleState"
  Switch1/1 -> Bus Creator1/20  "TireLoad"
  Rate Transition2/1 -> Switch/1
  Rate Transition1/1 -> Switch1/2, Switch/2
  Rate Transition3/1 -> Switch1/1
  Bus Selector1/18 -> Bus Creator1/18  "<RaceModeEnable>"

== system vd_controller_E9/021_SignalProcessing/213_PlausibiltyCheckandSignalMatching ==
  Bus_all : Inport
  9DFront_Plausibility : Subsystem
  9DRear_Plausibility : Subsystem
  Bus Creator1 : BusCreator  Inputs=22
  Bus Selector : BusSelector  OutputSignals=disable9Drear
  Bus Selector1 : BusSelector  OutputSignals=9DFront,9DRear,Settings,v2oVelocity,WheelSpeed,Suspension,Electric,WheelTorque,WheelAngle,DriverInput,DrivingMode,MotorTemp,InverterTemp,MotorSpeed,DriverRequest,DriverDemand,VD_Diag_z,TorqueOut_raw_z,RaceModeEnable
  DriverInput : Subsystem
  DriverRequest_Plausibility : Subsystem
  Electric_Plausibility : Subsystem
  InverterTemp_Plausibility : Subsystem
  MotorSpeed_Plausibility : Subsystem
  MotorTemp_Plausibility : Subsystem
  Suspension_Plausibility : Subsystem
  WheelSpeed_Plausibility : Subsystem
  v2oVelocity_Plausibility : Subsystem
  Bus_SignalProcessing : Outport
  wires:
  Bus Selector1/5 -> WheelSpeed_Plausibility/1(In)  "<WheelSpeed>"
  Bus Selector1/4 -> v2oVelocity_Plausibility/1(In)  "<v2oVelocity>"
  Bus_all/1 -> Bus Selector1/1
  Bus Selector1/8 -> Bus Creator1/9  "<WheelTorque>"
  Bus Creator1/1 -> Bus_SignalProcessing/1  "Bus_all"
  Bus Selector1/2 -> 9DRear_Plausibility/1(In)  "<9DRear>"
  Bus Selector1/6 -> Suspension_Plausibility/1(In)  "<Suspension>"
  Bus Selector1/7 -> Electric_Plausibility/1(In)  "<Electric>"
  Bus Selector1/9 -> Bus Creator1/10  "<WheelAngle>"
  Bus Selector1/3 -> Bus Selector/1, Bus Creator1/3  "<Settings>"
  Bus Selector1/10 -> DriverInput/1(DriverInput_in)  "<DriverInput>"
  Bus Selector1/12 -> MotorTemp_Plausibility/1(In)  "<MotorTemp>"
  Bus Selector1/14 -> MotorSpeed_Plausibility/1(In)  "<MotorSpeed>"
  Bus Selector1/15 -> DriverRequest_Plausibility/1(In)  "<DriverRequest>"
  Bus Selector1/1 -> 9DFront_Plausibility/1(In)  "<9DFront>"
  9DFront_Plausibility/1(9DFrontPlausible) -> Bus Creator1/1  "9DFront"
  9DRear_Plausibility/1(9DRearPlausible) -> Bus Creator1/2  "9DRear"
  v2oVelocity_Plausibility/1(v2oVelocityPlausible) -> Bus Creator1/4  "v2oVelocity"
  WheelSpeed_Plausibility/1(WheelSpeedPlausible) -> Bus Creator1/5  "WheelSpeed"
  Suspension_Plausibility/1(SuspensionPlausible) -> Bus Creator1/7  "Suspension"
  MotorSpeed_Plausibility/1(MotorSpeed) -> Bus Creator1/16  "MotorSpeed"
  Bus Selector1/13 -> InverterTemp_Plausibility/1(In)  "<InverterTemp>"
  DriverRequest_Plausibility/1(DriverRequest) -> Bus Creator1/18  "DriverRequest"
  Electric_Plausibility/1(ElectricPlausible) -> Bus Creator1/8  "Electric"
  WheelSpeed_Plausibility/2(WheelSpeed_Sq) -> Bus Creator1/6  "WheelSpeed_Sq"
  MotorSpeed_Plausibility/2(MotorSpeed_Sq) -> Bus Creator1/17  "MotorSpeed_Sq"
  DriverInput/1(DriverInput) -> Bus Creator1/11  "DriverInput"
  Bus Selector1/11 -> DriverInput/2(DrivingMode)  "<DrivingMode>"
  MotorTemp_Plausibility/1(MotorTempPlausible) -> Bus Creator1/12  "MotorTemp"
  MotorTemp_Plausibility/2(MotorTemp_Sq) -> Bus Creator1/13  "MotorTemp_Sq"
  InverterTemp_Plausibility/1(InverterTempPlausible) -> Bus Creator1/14  "InverterTemp"
  InverterTemp_Plausibility/2(InverterTemp_Sq) -> Bus Creator1/15  "InverterTemp_Sq"
  Bus Selector/1 -> 9DRear_Plausibility/2(In2)  "<disable9Drear>"
  Bus Selector1/16 -> Bus Creator1/19  "<DriverDemand>"
  Bus Selector1/19 -> Bus Creator1/22  "<RaceModeEnable>"
  Bus Selector1/17 -> Bus Creator1/20  "<VD_Diag_z>"
  Bus Selector1/18 -> Bus Creator1/21  "<TorqueOut_raw_z>"

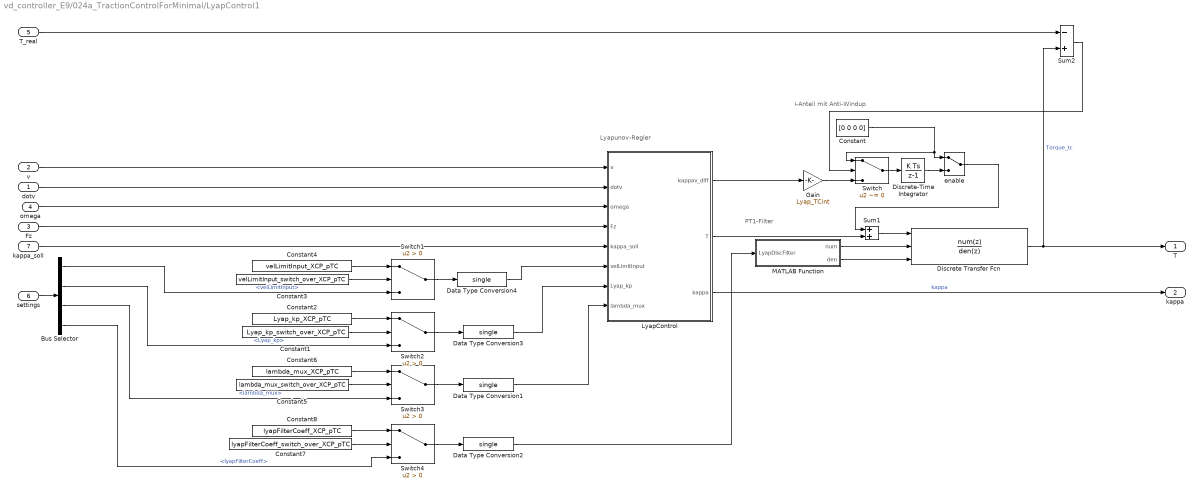
== system vd_controller_E9/024a_TractionControlForMinimal/LyapControl1 ==
  note: PT1-Filter
  note: Lyapunov-Regler
  note: I-Anteil mit Anti-Windup
  dotv : Inport
  v : Inport  Port=2
  Fz : Inport  Port=3
  omega : Inport  Port=4
  T_real : Inport  Port=5
  settings : Inport  Port=6
  kappa_soll : Inport  Port=7
  Bus Selector : BusSelector  OutputSignals=velLimitInput,Lyap_kp,lambda_mux,lyapFilterCoeff
  Constant : Constant  Value=[0 0 0 0]  OutDataTypeStr=Inherit: Inherit via back propagation
  Constant1 : Constant  Value=Lyap_kp_switch_over_XCP_pTC
  Constant2 : Constant  Value=Lyap_kp_XCP_pTC
  Constant3 : Constant  Value=velLimitInput_switch_over_XCP_pTC
  Constant4 : Constant  Value=velLimitInput_XCP_pTC  VectorParams1D=off
  Constant5 : Constant  Value=lambda_mux_switch_over_XCP_pTC
  Constant6 : Constant  Value=lambda_mux_XCP_pTC
  Constant7 : Constant  Value=lyapFilterCoeff_switch_over_XCP_pTC
  Constant8 : Constant  Value=lyapFilterCoeff_XCP_pTC
  Data Type Conversion{1..4} (4 alike) : DataTypeConversion  OutDataTypeStr=single
  Discrete Transfer Fcn : DiscreteTransferFcn  NumeratorSource=Input port  Numerator=1+LyapDiscFilter  DenominatorSource=Input port  Denominator=[1 LyapDiscFilter]  a0EqualsOne=on
      settings: InputPortMap=u0,p1,p3
  Discrete-Time Integrator : DiscreteIntegrator  InitialConditionSetting=State (most efficient)  SampleTime=-1  ICPrevOutput=DiscIntNeverNeededParam  ICPrevScaledInput=DiscIntNeverNeededParam
  Gain : Gain  Gain=Lyap_TCint
  LyapControl : MATLAB Function  TreatAsAtomicUnit=on  SystemSampleTime=0.001
  MATLAB Function : MATLAB Function  TreatAsAtomicUnit=on
  Sum1 : Sum
  Sum2 : Sum  Inputs=-+
  Switch : Switch  Criteria=u2 ~= 0
  Switch{1..4} (4 alike) : Switch  Criteria=u2 > Threshold
  enable : ManualSwitch
  T : Outport
  kappa : Outport  Port=2
  wires:
  T_real/1 -> Sum2/1
  Sum1/1 -> Discrete Transfer Fcn/1
  v/1 -> LyapControl/1(v)
  dotv/1 -> LyapControl/2(dotv)
  omega/1 -> LyapControl/3(omega)
  Fz/1 -> LyapControl/4(Fz)
  kappa_soll/1 -> LyapControl/5(kappa_soll)
  LyapControl/2(T) -> Sum1/2
  LyapControl/1(kappav_diff) -> Gain/1
  Discrete-Time Integrator/1 -> enable/2
  Constant/1 -> Switch/1, enable/1
  enable/1 -> Sum1/1
  LyapControl/3(kappa) -> kappa/1  "kappa"
  settings/1 -> Bus Selector/1
  Bus Selector/2 -> Switch2/3  "<Lyap_kp>"
  Discrete Transfer Fcn/1 -> Sum2/2, T/1  "Torque_tc"
  Switch/1 -> Discrete-Time Integrator/1
  Sum2/1 -> Switch/2
  Gain/1 -> Switch/3
  MATLAB Function/2(den) -> Discrete Transfer Fcn/3
  MATLAB Function/1(num) -> Discrete Transfer Fcn/2
  Bus Selector/1 -> Switch1/3  "<velLimitInput>"
  Bus Selector/4 -> Switch4/3  "<lyapFilterCoeff>"
  Bus Selector/3 -> Switch3/3  "<lambda_mux>"
  Constant3/1 -> Switch1/2
  Constant4/1 -> Switch1/1
  Constant2/1 -> Switch2/1
  Constant1/1 -> Switch2/2
  Constant6/1 -> Switch3/1
  Constant5/1 -> Switch3/2
  Constant8/1 -> Switch4/1
  Constant7/1 -> Switch4/2
  Switch1/1 -> Data Type Conversion4/1
  Switch2/1 -> Data Type Conversion3/1
  Switch3/1 -> Data Type Conversion1/1
  Switch4/1 -> Data Type Conversion2/1
  Data Type Conversion2/1 -> MATLAB Function/1(LyapDiscFilter)
  Data Type Conversion1/1 -> LyapControl/8(lambda_mux)
  Data Type Conversion3/1 -> LyapControl/7(Lyap_kp)
  Data Type Conversion4/1 -> LyapControl/6(velLimitInput)

== system vd_controller_E9/024a_TractionControlForMinimal/Schlupf Sollwert ==
  ConstSlipPercent : Inport
  "DriverDemand " : Inport  Port=2
  Gain : Gain  Gain=ones(4,1)
  Gain4 : Gain  Gain=-1*ones(4,1)
  Switch : Switch  Criteria=u2 > Threshold
  kappa_soll : Outport
  wires:
  Switch/1 -> kappa_soll/1
  ConstSlipPercent/1 -> Gain4/1, Gain/1
  Gain/1 -> Switch/1
  Gain4/1 -> Switch/3
  "DriverDemand "/1 -> Switch/2

== system vd_controller_E9/021_SignalProcessing/212_ManualMode/9DFront ==
  Signal_In : Inport
  Enable : Inport  Port=2
  Bitwise Operator : simulink/Logic and Bit Operations/Bitwise Operator  logicop=AND  UseBitMask=on  BitMask=bin2dec('11011001')  BitMaskRealWorld=Stored Integer
  Constant : Constant
  Constant1 : Constant
  Switch : Switch  Criteria=u2 ~= 0  Threshold=U2==0
  Terminator : Terminator
  9DFront : Outport
  wires:
  Bitwise Operator/1 -> Switch/2
  Signal_In/1 -> 9DFront/1  "9DFront"
  Enable/1 -> Bitwise Operator/1
  Constant/1 -> Switch/1
  Constant1/1 -> Switch/3
  Switch/1 -> Terminator/1  "9DFront"

== system vd_controller_E9/021_SignalProcessing/212_ManualMode/9DRear ==
  Signal_In : Inport
  Enable : Inport  Port=2
  Bitwise Operator : simulink/Logic and Bit Operations/Bitwise Operator  logicop=AND  UseBitMask=on  BitMask=bin2dec('11011001')  BitMaskRealWorld=Stored Integer
  Constant : Constant
  Constant1 : Constant
  Switch : Switch  Criteria=u2 ~= 0  Threshold=U2==0
  Terminator : Terminator
  9DRear : Outport
  wires:
  Enable/1 -> Bitwise Operator/1
  Signal_In/1 -> 9DRear/1  "9DRear"
  Bitwise Operator/1 -> Switch/2
  Constant/1 -> Switch/1
  Constant1/1 -> Switch/3
  Switch/1 -> Terminator/1  "9DRear"

== system vd_controller_E9/021_SignalProcessing/212_ManualMode/HMI_DriverNotice ==
  Signal_In : Inport
  Enable : Inport  Port=2
  Bitwise Operator : simulink/Logic and Bit Operations/Bitwise Operator  Commented=on  logicop=AND  UseBitMask=on  BitMask=bin2dec('11011001')  BitMaskRealWorld=Stored Integer
  Constant : Constant  Commented=on
  Switch : Switch  Commented=on  Criteria=u2 ~= 0  Threshold=U2==0
  Terminator : Terminator
  HMI_DriverNotice : Outport
  wires:
  Bitwise Operator/1 -> Switch/2
  Signal_In/1 -> HMI_DriverNotice/1  "HMI_DriverNotice"
  Enable/1 -> Bitwise Operator/1
  Constant/1 -> Switch/1
  Switch/1 -> Terminator/1  "HMI_DriverNotice"

== system vd_controller_E9/021_SignalProcessing/212_ManualMode/Subsystem17 ==
  Signal_In : Inport
  Enable : Inport  Port=2
  Bitwise Operator : simulink/Logic and Bit Operations/Bitwise Operator  logicop=AND  UseBitMask=on  BitMask=bin2dec('11011001')  BitMaskRealWorld=Stored Integer
  Constant : Constant
  Constant1 : Constant
  Switch : Switch  Criteria=u2 ~= 0  Threshold=U2==0
  Terminator : Terminator
  SP_DriverInput : Outport
  wires:
  Signal_In/1 -> SP_DriverInput/1
  Constant/1 -> Switch/1
  Constant1/1 -> Switch/3
  Bitwise Operator/1 -> Switch/2
  Enable/1 -> Bitwise Operator/1
  Switch/1 -> Terminator/1  "9DRear"

== system vd_controller_E9/021_SignalProcessing/212_ManualMode/electric ==
  Signal_In : Inport
  Enable : Inport  Port=2
  Bitwise Operator : simulink/Logic and Bit Operations/Bitwise Operator  logicop=AND  UseBitMask=on  BitMask=bin2dec('11011001')  BitMaskRealWorld=Stored Integer
  Constant : Constant
  Constant1 : Constant
  Switch : Switch  Criteria=u2 ~= 0  Threshold=U2==0
  Terminator : Terminator
  electric : Outport
  wires:
  Signal_In/1 -> electric/1  "electric"
  Bitwise Operator/1 -> Switch/2
  Enable/1 -> Bitwise Operator/1
  Constant1/1 -> Switch/3
  Switch/1 -> Terminator/1  "9DRear"
  Constant/1 -> Switch/1

== system vd_controller_E9/021_SignalProcessing/212_ManualMode/inverterTemp ==
  Signal_In : Inport
  Enable : Inport  Port=2
  Bitwise Operator : simulink/Logic and Bit Operations/Bitwise Operator  logicop=AND  UseBitMask=on  BitMask=bin2dec('11011001')  BitMaskRealWorld=Stored Integer
  Constant : Constant  OutDataTypeStr=single
  Switch : Switch  Criteria=u2 ~= 0  Threshold=U2==0  OutDataTypeStr=single
  inverterTemp : Outport  OutDataTypeStr=single  PortDimensions=4
  wires:
  Signal_In/1 -> Switch/3
  Enable/1 -> Bitwise Operator/1
  Switch/1 -> inverterTemp/1  "inverterTemp"
  Bitwise Operator/1 -> Switch/2
  Constant/1 -> Switch/1

== system vd_controller_E9/021_SignalProcessing/212_ManualMode/motorSpeed ==
  Signal_In : Inport
  Enable : Inport  Port=2
  Bitwise Operator : simulink/Logic and Bit Operations/Bitwise Operator  logicop=AND  UseBitMask=on  BitMask=bin2dec('11011001')  BitMaskRealWorld=Stored Integer
  Constant : Constant
  Switch : Switch  Criteria=u2 ~= 0  Threshold=U2==0
  motorSpeed : Outport
  wires:
  Bitwise Operator/1 -> Switch/2
  Switch/1 -> motorSpeed/1  "motorSpeed"
  Enable/1 -> Bitwise Operator/1
  Signal_In/1 -> Switch/3
  Constant/1 -> Switch/1

== system vd_controller_E9/021_SignalProcessing/212_ManualMode/motorTemp ==
  Signal_In : Inport
  Enable : Inport  Port=2
  Bitwise Operator : simulink/Logic and Bit Operations/Bitwise Operator  logicop=AND  UseBitMask=on  BitMask=bin2dec('11011001')  BitMaskRealWorld=Stored Integer
  Constant : Constant  OutDataTypeStr=single
  Switch : Switch  Criteria=u2 ~= 0  Threshold=U2==0  OutDataTypeStr=single
  motorTemp : Outport  OutDataTypeStr=single  PortDimensions=4
  wires:
  Bitwise Operator/1 -> Switch/2
  Switch/1 -> motorTemp/1  "motorTemp"
  Enable/1 -> Bitwise Operator/1
  Signal_In/1 -> Switch/3
  Constant/1 -> Switch/1

== system vd_controller_E9/021_SignalProcessing/212_ManualMode/settings ==
  Signal_In : Inport
  Enable : Inport  Port=2
  Bitwise Operator : simulink/Logic and Bit Operations/Bitwise Operator  logicop=AND  UseBitMask=on  BitMask=bin2dec('11011001')  BitMaskRealWorld=Stored Integer
  Constant : Constant
  Constant1 : Constant
  Switch : Switch  Criteria=u2 ~= 0  Threshold=U2==0
  Terminator : Terminator
  settings : Outport
  wires:
  Bitwise Operator/1 -> Switch/2
  Signal_In/1 -> settings/1  "settings"
  Enable/1 -> Bitwise Operator/1
  Constant1/1 -> Switch/3
  Constant/1 -> Switch/1
  Switch/1 -> Terminator/1  "settings"

== system vd_controller_E9/021_SignalProcessing/212_ManualMode/suspHall ==
  Signal_In : Inport
  Enable : Inport  Port=2
  Bitwise Operator : simulink/Logic and Bit Operations/Bitwise Operator  logicop=AND  UseBitMask=on  BitMask=bin2dec('11011001')  BitMaskRealWorld=Stored Integer
  Constant : Constant
  Constant1 : Constant
  Switch : Switch  Criteria=u2 ~= 0  Threshold=U2==0
  Terminator : Terminator
  suspHall : Outport
  wires:
  Signal_In/1 -> suspHall/1
  Constant1/1 -> Switch/3
  Enable/1 -> Bitwise Operator/1
  Switch/1 -> Terminator/1  "9DRear"
  Bitwise Operator/1 -> Switch/2
  Constant/1 -> Switch/1

== system vd_controller_E9/021_SignalProcessing/212_ManualMode/v2oVelocity ==
  Signal_In : Inport
  Enable : Inport  Port=2
  Bitwise Operator : simulink/Logic and Bit Operations/Bitwise Operator  logicop=AND  UseBitMask=on  BitMask=bin2dec('11011001')  BitMaskRealWorld=Stored Integer
  Constant : Constant
  Constant1 : Constant
  Switch : Switch  Criteria=u2 ~= 0  Threshold=U2==0
  Terminator : Terminator
  v2oVelocity : Outport
  wires:
  Signal_In/1 -> v2oVelocity/1  "v2oVelocity"
  Constant1/1 -> Switch/3
  Enable/1 -> Bitwise Operator/1
  Switch/1 -> Terminator/1  "9DRear"
  Bitwise Operator/1 -> Switch/2
  Constant/1 -> Switch/1

== system vd_controller_E9/021_SignalProcessing/212_ManualMode/wheelAngle ==
  Signal_In : Inport
  Enable : Inport  Port=2
  Bitwise Operator : simulink/Logic and Bit Operations/Bitwise Operator  logicop=AND  UseBitMask=on  BitMask=bin2dec('11011001')  BitMaskRealWorld=Stored Integer
  Constant : Constant
  Constant1 : Constant
  Switch : Switch  Criteria=u2 ~= 0  Threshold=U2==0
  Terminator : Terminator
  wheelAngle : Outport
  wires:
  Signal_In/1 -> wheelAngle/1
  Constant/1 -> Switch/1
  Constant1/1 -> Switch/3
  Bitwise Operator/1 -> Switch/2
  Enable/1 -> Bitwise Operator/1
  Switch/1 -> Terminator/1  "9DRear"

== system vd_controller_E9/021_SignalProcessing/212_ManualMode/wheelSpeed ==
  Signal_In : Inport
  Enable : Inport  Port=2
  Bitwise Operator : simulink/Logic and Bit Operations/Bitwise Operator  logicop=AND  UseBitMask=on  BitMask=bin2dec('11011001')  BitMaskRealWorld=Stored Integer
  Constant : Constant
  Constant1 : Constant
  Switch : Switch  Criteria=u2 ~= 0  Threshold=U2==0
  Terminator : Terminator
  wheelSpeed : Outport
  wires:
  Signal_In/1 -> wheelSpeed/1  "wheelSpeed"
  Constant1/1 -> Switch/3
  Enable/1 -> Bitwise Operator/1
  Switch/1 -> Terminator/1  "9DRear"
  Bitwise Operator/1 -> Switch/2
  Constant/1 -> Switch/1

== system vd_controller_E9/021_SignalProcessing/212_ManualMode/wheelTorque ==
  Signal_In : Inport
  Enable : Inport  Port=2
  Bitwise Operator : simulink/Logic and Bit Operations/Bitwise Operator  logicop=AND  UseBitMask=on  BitMask=bin2dec('11011001')  BitMaskRealWorld=Stored Integer
  Constant : Constant
  Constant1 : Constant
  Switch : Switch  Criteria=u2 ~= 0  Threshold=U2==0
  Terminator : Terminator
  wheelTorque : Outport
  wires:
  Signal_In/1 -> wheelTorque/1
  Constant/1 -> Switch/1
  Constant1/1 -> Switch/3
  Bitwise Operator/1 -> Switch/2
  Enable/1 -> Bitwise Operator/1
  Switch/1 -> Terminator/1  "9DRear"
